simulink model "Electrical_System_2018b_obfs"  (R2019b)
settings: Solver=VariableStepAuto  StartTime=0.0  StopTime=5  RelTol=1e-3  AbsTol=1e-3  EnableMultiTasking=on
InitFcn:
  | Steady_State_Initialisation;
StopFcn:
  | %sscexplore(simlog);
  | %Logging
undefined symbols (not defined in the file): abrlhklxvp, aexgmhuedq, afmfmjnutg, afpphrjpnc, ahuxbyvruc, alarvljztt, amxnyqmnuw, aodrlwvqie, aolhmuplyq, aqpmguuqkg, auesgwirzl, aurophlnng, awamelrhru, ayfhvxflxn, azxkacuhqc, babszerikg, bawhdqanwq, bevoqecvei, bltjvqbchx, bmqsuewujl, bsmyqjfgnf, btvjbsmnve, bywgxqeadw, bziaduxaer, bzmcmdqocb, bzsvyvetat, ccsjnrbsih, cdvenygxwh, cedkrnslhx, cjheorclzs, cjrdshrtqx, ckhavyhcza, ckxewznhlz, cmrcgyiplk, conenicnws, cqkejbgjnn, csfnuwymhe, cunupkhwbh, cwzfvzuxxh, dcadmadufn, dcfponivnv, ddtrqjrhjn, dfhoxvkqas, dfrhtcwpne, dfvomcagjv, djijwylxea, dnmeqksrrm, dnzewbdkaa, dsqcykyxav, dtswwlttmm, ecumpidjtv, edegaywrct, ejjjsmnejc, eknqnehjdz, emvdetzouf, esxbqkbahr, etnkkbreiq, eunoiiiirw, ewewcuedir, fatkfxdhtc ... (+386)
libraries: fl_lib x802, ee_lib x362, fl_ps_legacy_lib x160, nesl_utility x85
(part 25 of 26)

== system Electrical_System_2018b_obfs/Redacted_1221/Redacted_7996/Redacted_1/Redacted_4377/Redacted_6082/Redacted_4413/Positive_Neutral ==
  Open Circuit : fl_lib/Electrical/Electrical Elements/Open Circuit  v_specify=off  v_priority=None  v=0 V  v_nominal_specify=off  v_nominal_unit=V  v_nominal_value=1
      settings: SourceProductName=Simscape  SourceProductBaseCode=SS
  Redacted_9976 : PMIOPort  Side=Left
  Redacted_5180 : PMIOPort  Port=2  Side=Left
  Redacted_6712 : PMIOPort  Port=3  Side=Left
  Redacted_6595 : PMIOPort  Port=4  Side=Right
  Redacted_8408 : PMIOPort  Port=5  Side=Right
  connections:
  Open Circuit/LConn1 -- Redacted_6712/RConn1
  Redacted_6595/RConn1 -- Redacted_9976/RConn1
  Redacted_5180/RConn1 -- Redacted_8408/RConn1

== system Electrical_System_2018b_obfs/Redacted_1221/Redacted_7996/Redacted_1/Redacted_4377/Redacted_6082/Redacted_4413/Redacted_6190 ==
  Redacted_6825 : fl_lib/Electrical/Electrical Elements/Open Circuit  v_specify=off  v_priority=None  v=nafaxblafc V  v_nominal_specify=off  v_nominal_unit=V  v_nominal_value=uctqgjleyg
      settings: SourceProductName=Simscape  SourceProductBaseCode=SS
  Redacted_9976 : PMIOPort  Side=Left
  Redacted_5180 : PMIOPort  Port=2  Side=Left
  Redacted_6712 : PMIOPort  Port=3  Side=Left
  Redacted_6595 : PMIOPort  Port=4  Side=Right
  Redacted_8408 : PMIOPort  Port=5  Side=Right
  connections:
  Redacted_6825/LConn1 -- Redacted_5180/RConn1
  Redacted_6595/RConn1 -- Redacted_9976/RConn1
  Redacted_8408/RConn1 -- Redacted_6712/RConn1

== system Electrical_System_2018b_obfs/Redacted_1221/Redacted_7996/Redacted_1/Redacted_4377/Redacted_6082/Redacted_5550/Neutral_Negative ==
  Open Circuit : fl_lib/Electrical/Electrical Elements/Open Circuit  v_specify=off  v_priority=None  v=0 V  v_nominal_specify=off  v_nominal_unit=V  v_nominal_value=1
      settings: SourceProductName=Simscape  SourceProductBaseCode=SS
  Redacted_6826 : PMIOPort  Side=Left
  Redacted_51 : PMIOPort  Port=2  Side=Left
  Redacted_9515 : PMIOPort  Port=3  Side=Left
  Redacted_375 : PMIOPort  Port=4  Side=Right
  Redacted_6304 : PMIOPort  Port=5  Side=Right
  connections:
  Redacted_6304/RConn1 -- Redacted_9515/RConn1
  Open Circuit/LConn1 -- Redacted_6826/RConn1
  Redacted_51/RConn1 -- Redacted_375/RConn1

== system Electrical_System_2018b_obfs/Redacted_1221/Redacted_7996/Redacted_1/Redacted_4377/Redacted_6082/Redacted_5550/Positive_Neutral ==
  Open Circuit : fl_lib/Electrical/Electrical Elements/Open Circuit  v_specify=off  v_priority=None  v=0 V  v_nominal_specify=off  v_nominal_unit=V  v_nominal_value=1
      settings: SourceProductName=Simscape  SourceProductBaseCode=SS
  Redacted_6826 : PMIOPort  Side=Left
  Redacted_51 : PMIOPort  Port=2  Side=Left
  Redacted_9515 : PMIOPort  Port=3  Side=Left
  Redacted_375 : PMIOPort  Port=4  Side=Right
  Redacted_6304 : PMIOPort  Port=5  Side=Right
  connections:
  Open Circuit/LConn1 -- Redacted_9515/RConn1
  Redacted_375/RConn1 -- Redacted_6826/RConn1
  Redacted_51/RConn1 -- Redacted_6304/RConn1

== system Electrical_System_2018b_obfs/Redacted_1221/Redacted_7996/Redacted_1/Redacted_4377/Redacted_6082/Redacted_5550/Redacted_2952 ==
  Redacted_9904 : fl_lib/Electrical/Electrical Elements/Open Circuit  v_specify=off  v_priority=None  v=cbwtykvznf V  v_nominal_specify=off  v_nominal_unit=V  v_nominal_value=bbwdbtprkb
      settings: SourceProductName=Simscape  SourceProductBaseCode=SS
  Redacted_6826 : PMIOPort  Side=Left
  Redacted_51 : PMIOPort  Port=2  Side=Left
  Redacted_9515 : PMIOPort  Port=3  Side=Left
  Redacted_375 : PMIOPort  Port=4  Side=Right
  Redacted_6304 : PMIOPort  Port=5  Side=Right
  connections:
  Redacted_9904/LConn1 -- Redacted_51/RConn1
  Redacted_375/RConn1 -- Redacted_6826/RConn1
  Redacted_6304/RConn1 -- Redacted_9515/RConn1

== system Electrical_System_2018b_obfs/Redacted_1221/Redacted_7996/Redacted_1/Redacted_4377/Redacted_6082/Redacted_5713/Neutral_Negative ==
  Open Circuit : fl_lib/Electrical/Electrical Elements/Open Circuit  v_specify=off  v_priority=None  v=0 V  v_nominal_specify=off  v_nominal_unit=V  v_nominal_value=1
      settings: SourceProductName=Simscape  SourceProductBaseCode=SS
  Redacted_6138 : PMIOPort  Side=Left
  Redacted_1431 : PMIOPort  Port=2  Side=Left
  Redacted_7946 : PMIOPort  Port=3  Side=Left
  Redacted_819 : PMIOPort  Port=4  Side=Right
  Redacted_4816 : PMIOPort  Port=5  Side=Right
  connections:
  Redacted_4816/RConn1 -- Redacted_7946/RConn1
  Open Circuit/LConn1 -- Redacted_6138/RConn1
  Redacted_1431/RConn1 -- Redacted_819/RConn1

== system Electrical_System_2018b_obfs/Redacted_1221/Redacted_7996/Redacted_1/Redacted_4377/Redacted_6082/Redacted_5713/Positive_Neutral ==
  Open Circuit : fl_lib/Electrical/Electrical Elements/Open Circuit  v_specify=off  v_priority=None  v=0 V  v_nominal_specify=off  v_nominal_unit=V  v_nominal_value=1
      settings: SourceProductName=Simscape  SourceProductBaseCode=SS
  Redacted_6138 : PMIOPort  Side=Left
  Redacted_1431 : PMIOPort  Port=2  Side=Left
  Redacted_7946 : PMIOPort  Port=3  Side=Left
  Redacted_819 : PMIOPort  Port=4  Side=Right
  Redacted_4816 : PMIOPort  Port=5  Side=Right
  connections:
  Open Circuit/LConn1 -- Redacted_7946/RConn1
  Redacted_819/RConn1 -- Redacted_6138/RConn1
  Redacted_1431/RConn1 -- Redacted_4816/RConn1

== system Electrical_System_2018b_obfs/Redacted_1221/Redacted_7996/Redacted_1/Redacted_4377/Redacted_6082/Redacted_5713/Redacted_1184 ==
  Redacted_2299 : fl_lib/Electrical/Electrical Elements/Open Circuit  v_specify=off  v_priority=None  v=tqpmitufxi V  v_nominal_specify=off  v_nominal_unit=V  v_nominal_value=nizvadugds
      settings: SourceProductName=Simscape  SourceProductBaseCode=SS
  Redacted_6138 : PMIOPort  Side=Left
  Redacted_1431 : PMIOPort  Port=2  Side=Left
  Redacted_7946 : PMIOPort  Port=3  Side=Left
  Redacted_819 : PMIOPort  Port=4  Side=Right
  Redacted_4816 : PMIOPort  Port=5  Side=Right
  connections:
  Redacted_2299/LConn1 -- Redacted_1431/RConn1
  Redacted_819/RConn1 -- Redacted_6138/RConn1
  Redacted_4816/RConn1 -- Redacted_7946/RConn1

== system Electrical_System_2018b_obfs/Redacted_1221/Redacted_7996/Redacted_1/Redacted_4377/Redacted_6082/Redacted_5976/Neutral_Negative ==
  Open Circuit : fl_lib/Electrical/Electrical Elements/Open Circuit  v_specify=off  v_priority=None  v=0 V  v_nominal_specify=off  v_nominal_unit=V  v_nominal_value=1
      settings: SourceProductName=Simscape  SourceProductBaseCode=SS
  Redacted_9241 : PMIOPort  Side=Left
  Redacted_5276 : PMIOPort  Port=2  Side=Left
  Redacted_2400 : PMIOPort  Port=3  Side=Left
  Redacted_5406 : PMIOPort  Port=4  Side=Right
  Redacted_1074 : PMIOPort  Port=5  Side=Right
  connections:
  Redacted_5276/RConn1 -- Redacted_5406/RConn1
  Open Circuit/LConn1 -- Redacted_9241/RConn1
  Redacted_1074/RConn1 -- Redacted_2400/RConn1

== system Electrical_System_2018b_obfs/Redacted_1221/Redacted_7996/Redacted_1/Redacted_4377/Redacted_6082/Redacted_5976/Positive_Neutral ==
  Open Circuit : fl_lib/Electrical/Electrical Elements/Open Circuit  v_specify=off  v_priority=None  v=0 V  v_nominal_specify=off  v_nominal_unit=V  v_nominal_value=1
      settings: SourceProductName=Simscape  SourceProductBaseCode=SS
  Redacted_9241 : PMIOPort  Side=Left
  Redacted_5276 : PMIOPort  Port=2  Side=Left
  Redacted_2400 : PMIOPort  Port=3  Side=Left
  Redacted_5406 : PMIOPort  Port=4  Side=Right
  Redacted_1074 : PMIOPort  Port=5  Side=Right
  connections:
  Redacted_5276/RConn1 -- Redacted_1074/RConn1
  Redacted_5406/RConn1 -- Redacted_9241/RConn1
  Open Circuit/LConn1 -- Redacted_2400/RConn1

== system Electrical_System_2018b_obfs/Redacted_1221/Redacted_7996/Redacted_1/Redacted_4377/Redacted_6082/Redacted_5976/Redacted_5620 ==
  Redacted_9178 : fl_lib/Electrical/Electrical Elements/Open Circuit  v_specify=off  v_priority=None  v=jhtpowznxh V  v_nominal_specify=off  v_nominal_unit=V  v_nominal_value=mubuuhzqmu
      settings: SourceProductName=Simscape  SourceProductBaseCode=SS
  Redacted_9241 : PMIOPort  Side=Left
  Redacted_5276 : PMIOPort  Port=2  Side=Left
  Redacted_2400 : PMIOPort  Port=3  Side=Left
  Redacted_5406 : PMIOPort  Port=4  Side=Right
  Redacted_1074 : PMIOPort  Port=5  Side=Right
  connections:
  Redacted_1074/RConn1 -- Redacted_2400/RConn1
  Redacted_5406/RConn1 -- Redacted_9241/RConn1
  Redacted_9178/LConn1 -- Redacted_5276/RConn1

== system Electrical_System_2018b_obfs/Redacted_1221/Redacted_7996/Redacted_1/Redacted_4377/Redacted_6082/Redacted_6424/Neutral_Negative ==
  Open Circuit : fl_lib/Electrical/Electrical Elements/Open Circuit  v_specify=off  v_priority=None  v=0 V  v_nominal_specify=off  v_nominal_unit=V  v_nominal_value=1
      settings: SourceProductName=Simscape  SourceProductBaseCode=SS
  Redacted_4582 : PMIOPort  Side=Left
  Redacted_1544 : PMIOPort  Port=2  Side=Left
  Redacted_1581 : PMIOPort  Port=3  Side=Left
  Redacted_1961 : PMIOPort  Port=4  Side=Right
  Redacted_7479 : PMIOPort  Port=5  Side=Right
  connections:
  Redacted_7479/RConn1 -- Redacted_1581/RConn1
  Open Circuit/LConn1 -- Redacted_4582/RConn1
  Redacted_1544/RConn1 -- Redacted_1961/RConn1

== system Electrical_System_2018b_obfs/Redacted_1221/Redacted_7996/Redacted_1/Redacted_4377/Redacted_6082/Redacted_6424/Positive_Neutral ==
  Open Circuit : fl_lib/Electrical/Electrical Elements/Open Circuit  v_specify=off  v_priority=None  v=0 V  v_nominal_specify=off  v_nominal_unit=V  v_nominal_value=1
      settings: SourceProductName=Simscape  SourceProductBaseCode=SS
  Redacted_4582 : PMIOPort  Side=Left
  Redacted_1544 : PMIOPort  Port=2  Side=Left
  Redacted_1581 : PMIOPort  Port=3  Side=Left
  Redacted_1961 : PMIOPort  Port=4  Side=Right
  Redacted_7479 : PMIOPort  Port=5  Side=Right
  connections:
  Open Circuit/LConn1 -- Redacted_1581/RConn1
  Redacted_1961/RConn1 -- Redacted_4582/RConn1
  Redacted_1544/RConn1 -- Redacted_7479/RConn1

== system Electrical_System_2018b_obfs/Redacted_1221/Redacted_7996/Redacted_1/Redacted_4377/Redacted_6082/Redacted_6424/Redacted_7805 ==
  Redacted_3936 : fl_lib/Electrical/Electrical Elements/Open Circuit  v_specify=off  v_priority=None  v=fjoxglgvhp V  v_nominal_specify=off  v_nominal_unit=V  v_nominal_value=omyuclhrqc
      settings: SourceProductName=Simscape  SourceProductBaseCode=SS
  Redacted_4582 : PMIOPort  Side=Left
  Redacted_1544 : PMIOPort  Port=2  Side=Left
  Redacted_1581 : PMIOPort  Port=3  Side=Left
  Redacted_1961 : PMIOPort  Port=4  Side=Right
  Redacted_7479 : PMIOPort  Port=5  Side=Right
  connections:
  Redacted_3936/LConn1 -- Redacted_1544/RConn1
  Redacted_1961/RConn1 -- Redacted_4582/RConn1
  Redacted_7479/RConn1 -- Redacted_1581/RConn1

== system Electrical_System_2018b_obfs/Redacted_1221/Redacted_7996/Redacted_1/Redacted_4377/Redacted_6082/Redacted_7051/Neutral_Negative ==
  Open Circuit : fl_lib/Electrical/Electrical Elements/Open Circuit  v_specify=off  v_priority=None  v=0 V  v_nominal_specify=off  v_nominal_unit=V  v_nominal_value=1
      settings: SourceProductName=Simscape  SourceProductBaseCode=SS
  Redacted_2697 : PMIOPort  Side=Left
  Redacted_1518 : PMIOPort  Port=2  Side=Left
  Redacted_2395 : PMIOPort  Port=3  Side=Left
  Redacted_3537 : PMIOPort  Port=4  Side=Right
  Redacted_8383 : PMIOPort  Port=5  Side=Right
  connections:
  Redacted_1518/RConn1 -- Redacted_3537/RConn1
  Open Circuit/LConn1 -- Redacted_2697/RConn1
  Redacted_8383/RConn1 -- Redacted_2395/RConn1

== system Electrical_System_2018b_obfs/Redacted_1221/Redacted_7996/Redacted_1/Redacted_4377/Redacted_6082/Redacted_7051/Positive_Neutral ==
  Open Circuit : fl_lib/Electrical/Electrical Elements/Open Circuit  v_specify=off  v_priority=None  v=0 V  v_nominal_specify=off  v_nominal_unit=V  v_nominal_value=1
      settings: SourceProductName=Simscape  SourceProductBaseCode=SS
  Redacted_2697 : PMIOPort  Side=Left
  Redacted_1518 : PMIOPort  Port=2  Side=Left
  Redacted_2395 : PMIOPort  Port=3  Side=Left
  Redacted_3537 : PMIOPort  Port=4  Side=Right
  Redacted_8383 : PMIOPort  Port=5  Side=Right
  connections:
  Redacted_1518/RConn1 -- Redacted_8383/RConn1
  Redacted_3537/RConn1 -- Redacted_2697/RConn1
  Open Circuit/LConn1 -- Redacted_2395/RConn1

== system Electrical_System_2018b_obfs/Redacted_1221/Redacted_7996/Redacted_1/Redacted_4377/Redacted_6082/Redacted_7051/Redacted_1021 ==
  Redacted_3666 : fl_lib/Electrical/Electrical Elements/Open Circuit  v_specify=off  v_priority=None  v=jitpzdpdri V  v_nominal_specify=off  v_nominal_unit=V  v_nominal_value=zhywmqlonq
      settings: SourceProductName=Simscape  SourceProductBaseCode=SS
  Redacted_2697 : PMIOPort  Side=Left
  Redacted_1518 : PMIOPort  Port=2  Side=Left
  Redacted_2395 : PMIOPort  Port=3  Side=Left
  Redacted_3537 : PMIOPort  Port=4  Side=Right
  Redacted_8383 : PMIOPort  Port=5  Side=Right
  connections:
  Redacted_8383/RConn1 -- Redacted_2395/RConn1
  Redacted_3537/RConn1 -- Redacted_2697/RConn1
  Redacted_3666/LConn1 -- Redacted_1518/RConn1

== system Electrical_System_2018b_obfs/Redacted_1221/Redacted_7996/Redacted_1/Redacted_4377/Redacted_6082/Redacted_7884/Neutral_Negative ==
  Open Circuit : fl_lib/Electrical/Electrical Elements/Open Circuit  v_specify=off  v_priority=None  v=0 V  v_nominal_specify=off  v_nominal_unit=V  v_nominal_value=1
      settings: SourceProductName=Simscape  SourceProductBaseCode=SS
  Redacted_6224 : PMIOPort  Side=Left
  Redacted_4321 : PMIOPort  Port=2  Side=Left
  Redacted_2243 : PMIOPort  Port=3  Side=Left
  Redacted_707 : PMIOPort  Port=4  Side=Right
  Redacted_8636 : PMIOPort  Port=5  Side=Right
  connections:
  Redacted_4321/RConn1 -- Redacted_707/RConn1
  Open Circuit/LConn1 -- Redacted_6224/RConn1
  Redacted_8636/RConn1 -- Redacted_2243/RConn1

== system Electrical_System_2018b_obfs/Redacted_1221/Redacted_7996/Redacted_1/Redacted_4377/Redacted_6082/Redacted_7884/Positive_Neutral ==
  Open Circuit : fl_lib/Electrical/Electrical Elements/Open Circuit  v_specify=off  v_priority=None  v=0 V  v_nominal_specify=off  v_nominal_unit=V  v_nominal_value=1
      settings: SourceProductName=Simscape  SourceProductBaseCode=SS
  Redacted_6224 : PMIOPort  Side=Left
  Redacted_4321 : PMIOPort  Port=2  Side=Left
  Redacted_2243 : PMIOPort  Port=3  Side=Left
  Redacted_707 : PMIOPort  Port=4  Side=Right
  Redacted_8636 : PMIOPort  Port=5  Side=Right
  connections:
  Redacted_4321/RConn1 -- Redacted_8636/RConn1
  Redacted_707/RConn1 -- Redacted_6224/RConn1
  Open Circuit/LConn1 -- Redacted_2243/RConn1

== system Electrical_System_2018b_obfs/Redacted_1221/Redacted_7996/Redacted_1/Redacted_4377/Redacted_6082/Redacted_7884/Redacted_81 ==
  Redacted_8822 : fl_lib/Electrical/Electrical Elements/Open Circuit  v_specify=off  v_priority=None  v=nrbmgkomdb V  v_nominal_specify=off  v_nominal_unit=V  v_nominal_value=chrfcotgkg
      settings: SourceProductName=Simscape  SourceProductBaseCode=SS
  Redacted_6224 : PMIOPort  Side=Left
  Redacted_4321 : PMIOPort  Port=2  Side=Left
  Redacted_2243 : PMIOPort  Port=3  Side=Left
  Redacted_707 : PMIOPort  Port=4  Side=Right
  Redacted_8636 : PMIOPort  Port=5  Side=Right
  connections:
  Redacted_8636/RConn1 -- Redacted_2243/RConn1
  Redacted_707/RConn1 -- Redacted_6224/RConn1
  Redacted_8822/LConn1 -- Redacted_4321/RConn1

== system Electrical_System_2018b_obfs/Redacted_1221/Redacted_7996/Redacted_1/Redacted_4377/Redacted_6082/Redacted_8502/Neutral_Negative ==
  Open Circuit : fl_lib/Electrical/Electrical Elements/Open Circuit  v_specify=off  v_priority=None  v=0 V  v_nominal_specify=off  v_nominal_unit=V  v_nominal_value=1
      settings: SourceProductName=Simscape  SourceProductBaseCode=SS
  Redacted_389 : PMIOPort  Side=Left
  Redacted_6488 : PMIOPort  Port=2  Side=Left
  Redacted_5156 : PMIOPort  Port=3  Side=Left
  Redacted_180 : PMIOPort  Port=4  Side=Right
  Redacted_7018 : PMIOPort  Port=5  Side=Right
  connections:
  Redacted_6488/RConn1 -- Redacted_180/RConn1
  Open Circuit/LConn1 -- Redacted_389/RConn1
  Redacted_7018/RConn1 -- Redacted_5156/RConn1

== system Electrical_System_2018b_obfs/Redacted_1221/Redacted_7996/Redacted_1/Redacted_4377/Redacted_6082/Redacted_8502/Positive_Neutral ==
  Open Circuit : fl_lib/Electrical/Electrical Elements/Open Circuit  v_specify=off  v_priority=None  v=0 V  v_nominal_specify=off  v_nominal_unit=V  v_nominal_value=1
      settings: SourceProductName=Simscape  SourceProductBaseCode=SS
  Redacted_389 : PMIOPort  Side=Left
  Redacted_6488 : PMIOPort  Port=2  Side=Left
  Redacted_5156 : PMIOPort  Port=3  Side=Left
  Redacted_180 : PMIOPort  Port=4  Side=Right
  Redacted_7018 : PMIOPort  Port=5  Side=Right
  connections:
  Redacted_6488/RConn1 -- Redacted_7018/RConn1
  Redacted_180/RConn1 -- Redacted_389/RConn1
  Open Circuit/LConn1 -- Redacted_5156/RConn1

== system Electrical_System_2018b_obfs/Redacted_1221/Redacted_7996/Redacted_1/Redacted_4377/Redacted_6082/Redacted_8502/Redacted_4068 ==
  Redacted_9772 : fl_lib/Electrical/Electrical Elements/Open Circuit  v_specify=off  v_priority=None  v=truhycjrml V  v_nominal_specify=off  v_nominal_unit=V  v_nominal_value=fuzhyyoiey
      settings: SourceProductName=Simscape  SourceProductBaseCode=SS
  Redacted_389 : PMIOPort  Side=Left
  Redacted_6488 : PMIOPort  Port=2  Side=Left
  Redacted_5156 : PMIOPort  Port=3  Side=Left
  Redacted_180 : PMIOPort  Port=4  Side=Right
  Redacted_7018 : PMIOPort  Port=5  Side=Right
  connections:
  Redacted_7018/RConn1 -- Redacted_5156/RConn1
  Redacted_180/RConn1 -- Redacted_389/RConn1
  Redacted_9772/LConn1 -- Redacted_6488/RConn1

== system Electrical_System_2018b_obfs/Redacted_1221/Redacted_7996/Redacted_1/Redacted_4377/Redacted_6082/Redacted_9034/Neutral_Negative ==
  Open Circuit : fl_lib/Electrical/Electrical Elements/Open Circuit  v_specify=off  v_priority=None  v=0 V  v_nominal_specify=off  v_nominal_unit=V  v_nominal_value=1
      settings: SourceProductName=Simscape  SourceProductBaseCode=SS
  Redacted_4887 : PMIOPort  Side=Left
  Redacted_5529 : PMIOPort  Port=2  Side=Left
  Redacted_4069 : PMIOPort  Port=3  Side=Left
  Redacted_1826 : PMIOPort  Port=4  Side=Right
  Redacted_1222 : PMIOPort  Port=5  Side=Right
  connections:
  Redacted_1222/RConn1 -- Redacted_4069/RConn1
  Open Circuit/LConn1 -- Redacted_4887/RConn1
  Redacted_5529/RConn1 -- Redacted_1826/RConn1

== system Electrical_System_2018b_obfs/Redacted_1221/Redacted_7996/Redacted_1/Redacted_4377/Redacted_6082/Redacted_9034/Positive_Neutral ==
  Open Circuit : fl_lib/Electrical/Electrical Elements/Open Circuit  v_specify=off  v_priority=None  v=0 V  v_nominal_specify=off  v_nominal_unit=V  v_nominal_value=1
      settings: SourceProductName=Simscape  SourceProductBaseCode=SS
  Redacted_4887 : PMIOPort  Side=Left
  Redacted_5529 : PMIOPort  Port=2  Side=Left
  Redacted_4069 : PMIOPort  Port=3  Side=Left
  Redacted_1826 : PMIOPort  Port=4  Side=Right
  Redacted_1222 : PMIOPort  Port=5  Side=Right
  connections:
  Open Circuit/LConn1 -- Redacted_4069/RConn1
  Redacted_1826/RConn1 -- Redacted_4887/RConn1
  Redacted_5529/RConn1 -- Redacted_1222/RConn1

== system Electrical_System_2018b_obfs/Redacted_1221/Redacted_7996/Redacted_1/Redacted_4377/Redacted_6082/Redacted_9034/Redacted_4182 ==
  Redacted_1436 : fl_lib/Electrical/Electrical Elements/Open Circuit  v_specify=off  v_priority=None  v=zzrofiuybt V  v_nominal_specify=off  v_nominal_unit=V  v_nominal_value=ignlzzzuid
      settings: SourceProductName=Simscape  SourceProductBaseCode=SS
  Redacted_4887 : PMIOPort  Side=Left
  Redacted_5529 : PMIOPort  Port=2  Side=Left
  Redacted_4069 : PMIOPort  Port=3  Side=Left
  Redacted_1826 : PMIOPort  Port=4  Side=Right
  Redacted_1222 : PMIOPort  Port=5  Side=Right
  connections:
  Redacted_1436/LConn1 -- Redacted_5529/RConn1
  Redacted_1826/RConn1 -- Redacted_4887/RConn1
  Redacted_1222/RConn1 -- Redacted_4069/RConn1

== system Electrical_System_2018b_obfs/Redacted_1221/Redacted_7996/Redacted_1/Redacted_4377/Redacted_6082/Redacted_9572/Neutral_Negative ==
  Open Circuit : fl_lib/Electrical/Electrical Elements/Open Circuit  v_specify=off  v_priority=None  v=0 V  v_nominal_specify=off  v_nominal_unit=V  v_nominal_value=1
      settings: SourceProductName=Simscape  SourceProductBaseCode=SS
  Redacted_435 : PMIOPort  Side=Left
  Redacted_1376 : PMIOPort  Port=2  Side=Left
  Redacted_8237 : PMIOPort  Port=3  Side=Left
  Redacted_4941 : PMIOPort  Port=4  Side=Right
  Redacted_729 : PMIOPort  Port=5  Side=Right
  connections:
  Redacted_1376/RConn1 -- Redacted_4941/RConn1
  Open Circuit/LConn1 -- Redacted_435/RConn1
  Redacted_729/RConn1 -- Redacted_8237/RConn1

== system Electrical_System_2018b_obfs/Redacted_1221/Redacted_7996/Redacted_1/Redacted_4377/Redacted_6082/Redacted_9572/Positive_Neutral ==
  Open Circuit : fl_lib/Electrical/Electrical Elements/Open Circuit  v_specify=off  v_priority=None  v=0 V  v_nominal_specify=off  v_nominal_unit=V  v_nominal_value=1
      settings: SourceProductName=Simscape  SourceProductBaseCode=SS
  Redacted_435 : PMIOPort  Side=Left
  Redacted_1376 : PMIOPort  Port=2  Side=Left
  Redacted_8237 : PMIOPort  Port=3  Side=Left
  Redacted_4941 : PMIOPort  Port=4  Side=Right
  Redacted_729 : PMIOPort  Port=5  Side=Right
  connections:
  Redacted_1376/RConn1 -- Redacted_729/RConn1
  Redacted_4941/RConn1 -- Redacted_435/RConn1
  Open Circuit/LConn1 -- Redacted_8237/RConn1

== system Electrical_System_2018b_obfs/Redacted_1221/Redacted_7996/Redacted_1/Redacted_4377/Redacted_6082/Redacted_9572/Redacted_3288 ==
  Redacted_4505 : fl_lib/Electrical/Electrical Elements/Open Circuit  v_specify=off  v_priority=None  v=bjybeoqvmc V  v_nominal_specify=off  v_nominal_unit=V  v_nominal_value=ldxcbaigcw
      settings: SourceProductName=Simscape  SourceProductBaseCode=SS
  Redacted_435 : PMIOPort  Side=Left
  Redacted_1376 : PMIOPort  Port=2  Side=Left
  Redacted_8237 : PMIOPort  Port=3  Side=Left
  Redacted_4941 : PMIOPort  Port=4  Side=Right
  Redacted_729 : PMIOPort  Port=5  Side=Right
  connections:
  Redacted_729/RConn1 -- Redacted_8237/RConn1
  Redacted_4941/RConn1 -- Redacted_435/RConn1
  Redacted_4505/LConn1 -- Redacted_1376/RConn1

== system Electrical_System_2018b_obfs/Redacted_1221/Redacted_7996/Redacted_1/Redacted_4377/Redacted_6082/Redacted_980/Neutral_Negative ==
  Open Circuit : fl_lib/Electrical/Electrical Elements/Open Circuit  v_specify=off  v_priority=None  v=0 V  v_nominal_specify=off  v_nominal_unit=V  v_nominal_value=1
      settings: SourceProductName=Simscape  SourceProductBaseCode=SS
  Redacted_3281 : PMIOPort  Side=Left
  Redacted_9175 : PMIOPort  Port=2  Side=Left
  Redacted_1087 : PMIOPort  Port=3  Side=Left
  Redacted_2672 : PMIOPort  Port=4  Side=Right
  Redacted_3599 : PMIOPort  Port=5  Side=Right
  connections:
  Redacted_3599/RConn1 -- Redacted_1087/RConn1
  Open Circuit/LConn1 -- Redacted_3281/RConn1
  Redacted_9175/RConn1 -- Redacted_2672/RConn1

== system Electrical_System_2018b_obfs/Redacted_1221/Redacted_7996/Redacted_1/Redacted_4377/Redacted_6082/Redacted_980/Positive_Neutral ==
  Open Circuit : fl_lib/Electrical/Electrical Elements/Open Circuit  v_specify=off  v_priority=None  v=0 V  v_nominal_specify=off  v_nominal_unit=V  v_nominal_value=1
      settings: SourceProductName=Simscape  SourceProductBaseCode=SS
  Redacted_3281 : PMIOPort  Side=Left
  Redacted_9175 : PMIOPort  Port=2  Side=Left
  Redacted_1087 : PMIOPort  Port=3  Side=Left
  Redacted_2672 : PMIOPort  Port=4  Side=Right
  Redacted_3599 : PMIOPort  Port=5  Side=Right
  connections:
  Open Circuit/LConn1 -- Redacted_1087/RConn1
  Redacted_2672/RConn1 -- Redacted_3281/RConn1
  Redacted_9175/RConn1 -- Redacted_3599/RConn1

== system Electrical_System_2018b_obfs/Redacted_1221/Redacted_7996/Redacted_1/Redacted_4377/Redacted_6082/Redacted_980/Redacted_8833 ==
  Redacted_4926 : fl_lib/Electrical/Electrical Elements/Open Circuit  v_specify=off  v_priority=None  v=pdiyatassn V  v_nominal_specify=off  v_nominal_unit=V  v_nominal_value=uflvhyhiqw
      settings: SourceProductName=Simscape  SourceProductBaseCode=SS
  Redacted_3281 : PMIOPort  Side=Left
  Redacted_9175 : PMIOPort  Port=2  Side=Left
  Redacted_1087 : PMIOPort  Port=3  Side=Left
  Redacted_2672 : PMIOPort  Port=4  Side=Right
  Redacted_3599 : PMIOPort  Port=5  Side=Right
  connections:
  Redacted_4926/LConn1 -- Redacted_9175/RConn1
  Redacted_2672/RConn1 -- Redacted_3281/RConn1
  Redacted_3599/RConn1 -- Redacted_1087/RConn1

== system Electrical_System_2018b_obfs/Redacted_1221/Redacted_7996/Redacted_2/Redacted_38/Redacted_8107/Redacted_3070/Neutral_Negative ==
  Open Circuit : fl_lib/Electrical/Electrical Elements/Open Circuit  v_specify=off  v_priority=None  v=0 V  v_nominal_specify=off  v_nominal_unit=V  v_nominal_value=1
      settings: SourceProductName=Simscape  SourceProductBaseCode=SS
  Redacted_9800 : PMIOPort  Side=Left
  Redacted_6600 : PMIOPort  Port=2  Side=Left
  Redacted_5239 : PMIOPort  Port=3  Side=Left
  Redacted_3081 : PMIOPort  Port=4  Side=Right
  Redacted_7642 : PMIOPort  Port=5  Side=Right
  connections:
  Redacted_7642/RConn1 -- Redacted_5239/RConn1
  Open Circuit/LConn1 -- Redacted_9800/RConn1
  Redacted_6600/RConn1 -- Redacted_3081/RConn1

== system Electrical_System_2018b_obfs/Redacted_1221/Redacted_7996/Redacted_2/Redacted_38/Redacted_8107/Redacted_3070/Positive_Neutral ==
  Open Circuit : fl_lib/Electrical/Electrical Elements/Open Circuit  v_specify=off  v_priority=None  v=0 V  v_nominal_specify=off  v_nominal_unit=V  v_nominal_value=1
      settings: SourceProductName=Simscape  SourceProductBaseCode=SS
  Redacted_9800 : PMIOPort  Side=Left
  Redacted_6600 : PMIOPort  Port=2  Side=Left
  Redacted_5239 : PMIOPort  Port=3  Side=Left
  Redacted_3081 : PMIOPort  Port=4  Side=Right
  Redacted_7642 : PMIOPort  Port=5  Side=Right
  connections:
  Open Circuit/LConn1 -- Redacted_5239/RConn1
  Redacted_3081/RConn1 -- Redacted_9800/RConn1
  Redacted_6600/RConn1 -- Redacted_7642/RConn1

== system Electrical_System_2018b_obfs/Redacted_1221/Redacted_7996/Redacted_2/Redacted_38/Redacted_8107/Redacted_3070/Redacted_6581 ==
  Redacted_9951 : fl_lib/Electrical/Electrical Elements/Open Circuit  v_specify=off  v_priority=None  v=kbecunztrl V  v_nominal_specify=off  v_nominal_unit=V  v_nominal_value=jkubweymaj
      settings: SourceProductName=Simscape  SourceProductBaseCode=SS
  Redacted_9800 : PMIOPort  Side=Left
  Redacted_6600 : PMIOPort  Port=2  Side=Left
  Redacted_5239 : PMIOPort  Port=3  Side=Left
  Redacted_3081 : PMIOPort  Port=4  Side=Right
  Redacted_7642 : PMIOPort  Port=5  Side=Right
  connections:
  Redacted_9951/LConn1 -- Redacted_6600/RConn1
  Redacted_3081/RConn1 -- Redacted_9800/RConn1
  Redacted_7642/RConn1 -- Redacted_5239/RConn1

== system Electrical_System_2018b_obfs/Redacted_1221/Redacted_7996/Redacted_2/Redacted_38/Redacted_8107/Redacted_8444/Neutral_Negative ==
  Open Circuit : fl_lib/Electrical/Electrical Elements/Open Circuit  v_specify=off  v_priority=None  v=0 V  v_nominal_specify=off  v_nominal_unit=V  v_nominal_value=1
      settings: SourceProductName=Simscape  SourceProductBaseCode=SS
  Redacted_8974 : PMIOPort  Side=Left
  Redacted_9727 : PMIOPort  Port=2  Side=Left
  Redacted_5818 : PMIOPort  Port=3  Side=Left
  Redacted_9930 : PMIOPort  Port=4  Side=Right
  Redacted_8840 : PMIOPort  Port=5  Side=Right
  connections:
  Redacted_9727/RConn1 -- Redacted_9930/RConn1
  Open Circuit/LConn1 -- Redacted_8974/RConn1
  Redacted_8840/RConn1 -- Redacted_5818/RConn1

== system Electrical_System_2018b_obfs/Redacted_1221/Redacted_7996/Redacted_2/Redacted_38/Redacted_8107/Redacted_8444/Positive_Neutral ==
  Open Circuit : fl_lib/Electrical/Electrical Elements/Open Circuit  v_specify=off  v_priority=None  v=0 V  v_nominal_specify=off  v_nominal_unit=V  v_nominal_value=1
      settings: SourceProductName=Simscape  SourceProductBaseCode=SS
  Redacted_8974 : PMIOPort  Side=Left
  Redacted_9727 : PMIOPort  Port=2  Side=Left
  Redacted_5818 : PMIOPort  Port=3  Side=Left
  Redacted_9930 : PMIOPort  Port=4  Side=Right
  Redacted_8840 : PMIOPort  Port=5  Side=Right
  connections:
  Redacted_9727/RConn1 -- Redacted_8840/RConn1
  Redacted_9930/RConn1 -- Redacted_8974/RConn1
  Open Circuit/LConn1 -- Redacted_5818/RConn1

== system Electrical_System_2018b_obfs/Redacted_1221/Redacted_7996/Redacted_2/Redacted_38/Redacted_8107/Redacted_8444/Redacted_3917 ==
  Redacted_1857 : fl_lib/Electrical/Electrical Elements/Open Circuit  v_specify=off  v_priority=None  v=xcvpklmsqm V  v_nominal_specify=off  v_nominal_unit=V  v_nominal_value=rzgrfophqu
      settings: SourceProductName=Simscape  SourceProductBaseCode=SS
  Redacted_8974 : PMIOPort  Side=Left
  Redacted_9727 : PMIOPort  Port=2  Side=Left
  Redacted_5818 : PMIOPort  Port=3  Side=Left
  Redacted_9930 : PMIOPort  Port=4  Side=Right
  Redacted_8840 : PMIOPort  Port=5  Side=Right
  connections:
  Redacted_8840/RConn1 -- Redacted_5818/RConn1
  Redacted_9930/RConn1 -- Redacted_8974/RConn1
  Redacted_1857/LConn1 -- Redacted_9727/RConn1

== system Electrical_System_2018b_obfs/Redacted_1221/Redacted_7996/Redacted_7418/Redacted_4377/Redacted_6082/Redacted_144/Neutral_Negative ==
  Open Circuit : fl_lib/Electrical/Electrical Elements/Open Circuit  v_specify=off  v_priority=None  v=0 V  v_nominal_specify=off  v_nominal_unit=V  v_nominal_value=1
      settings: SourceProductName=Simscape  SourceProductBaseCode=SS
  Redacted_3879 : PMIOPort  Side=Left
  Redacted_3368 : PMIOPort  Port=2  Side=Left
  Redacted_9451 : PMIOPort  Port=3  Side=Left
  Redacted_8432 : PMIOPort  Port=4  Side=Right
  Redacted_6806 : PMIOPort  Port=5  Side=Right
  connections:
  Redacted_6806/RConn1 -- Redacted_9451/RConn1
  Open Circuit/LConn1 -- Redacted_3879/RConn1
  Redacted_3368/RConn1 -- Redacted_8432/RConn1

== system Electrical_System_2018b_obfs/Redacted_1221/Redacted_7996/Redacted_7418/Redacted_4377/Redacted_6082/Redacted_144/Positive_Neutral ==
  Open Circuit : fl_lib/Electrical/Electrical Elements/Open Circuit  v_specify=off  v_priority=None  v=0 V  v_nominal_specify=off  v_nominal_unit=V  v_nominal_value=1
      settings: SourceProductName=Simscape  SourceProductBaseCode=SS
  Redacted_3879 : PMIOPort  Side=Left
  Redacted_3368 : PMIOPort  Port=2  Side=Left
  Redacted_9451 : PMIOPort  Port=3  Side=Left
  Redacted_8432 : PMIOPort  Port=4  Side=Right
  Redacted_6806 : PMIOPort  Port=5  Side=Right
  connections:
  Open Circuit/LConn1 -- Redacted_9451/RConn1
  Redacted_8432/RConn1 -- Redacted_3879/RConn1
  Redacted_3368/RConn1 -- Redacted_6806/RConn1

== system Electrical_System_2018b_obfs/Redacted_1221/Redacted_7996/Redacted_7418/Redacted_4377/Redacted_6082/Redacted_144/Redacted_9503 ==
  Redacted_4565 : fl_lib/Electrical/Electrical Elements/Open Circuit  v_specify=off  v_priority=None  v=skhzijqmdj V  v_nominal_specify=off  v_nominal_unit=V  v_nominal_value=jdqusxliha
      settings: SourceProductName=Simscape  SourceProductBaseCode=SS
  Redacted_3879 : PMIOPort  Side=Left
  Redacted_3368 : PMIOPort  Port=2  Side=Left
  Redacted_9451 : PMIOPort  Port=3  Side=Left
  Redacted_8432 : PMIOPort  Port=4  Side=Right
  Redacted_6806 : PMIOPort  Port=5  Side=Right
  connections:
  Redacted_4565/LConn1 -- Redacted_3368/RConn1
  Redacted_8432/RConn1 -- Redacted_3879/RConn1
  Redacted_6806/RConn1 -- Redacted_9451/RConn1

== system Electrical_System_2018b_obfs/Redacted_1221/Redacted_7996/Redacted_7418/Redacted_4377/Redacted_6082/Redacted_1544/Neutral_Negative ==
  Open Circuit : fl_lib/Electrical/Electrical Elements/Open Circuit  v_specify=off  v_priority=None  v=0 V  v_nominal_specify=off  v_nominal_unit=V  v_nominal_value=1
      settings: SourceProductName=Simscape  SourceProductBaseCode=SS
  Redacted_697 : PMIOPort  Side=Left
  Redacted_9789 : PMIOPort  Port=2  Side=Left
  Redacted_5820 : PMIOPort  Port=3  Side=Left
  Redacted_1167 : PMIOPort  Port=4  Side=Right
  Redacted_9408 : PMIOPort  Port=5  Side=Right
  connections:
  Redacted_9408/RConn1 -- Redacted_5820/RConn1
  Open Circuit/LConn1 -- Redacted_697/RConn1
  Redacted_9789/RConn1 -- Redacted_1167/RConn1

== system Electrical_System_2018b_obfs/Redacted_1221/Redacted_7996/Redacted_7418/Redacted_4377/Redacted_6082/Redacted_1544/Positive_Neutral ==
  Open Circuit : fl_lib/Electrical/Electrical Elements/Open Circuit  v_specify=off  v_priority=None  v=0 V  v_nominal_specify=off  v_nominal_unit=V  v_nominal_value=1
      settings: SourceProductName=Simscape  SourceProductBaseCode=SS
  Redacted_697 : PMIOPort  Side=Left
  Redacted_9789 : PMIOPort  Port=2  Side=Left
  Redacted_5820 : PMIOPort  Port=3  Side=Left
  Redacted_1167 : PMIOPort  Port=4  Side=Right
  Redacted_9408 : PMIOPort  Port=5  Side=Right
  connections:
  Open Circuit/LConn1 -- Redacted_5820/RConn1
  Redacted_1167/RConn1 -- Redacted_697/RConn1
  Redacted_9789/RConn1 -- Redacted_9408/RConn1

== system Electrical_System_2018b_obfs/Redacted_1221/Redacted_7996/Redacted_7418/Redacted_4377/Redacted_6082/Redacted_1544/Redacted_4672 ==
  Redacted_7052 : fl_lib/Electrical/Electrical Elements/Open Circuit  v_specify=off  v_priority=None  v=fpovqwbuex V  v_nominal_specify=off  v_nominal_unit=V  v_nominal_value=qdnyfekgsz
      settings: SourceProductName=Simscape  SourceProductBaseCode=SS
  Redacted_697 : PMIOPort  Side=Left
  Redacted_9789 : PMIOPort  Port=2  Side=Left
  Redacted_5820 : PMIOPort  Port=3  Side=Left
  Redacted_1167 : PMIOPort  Port=4  Side=Right
  Redacted_9408 : PMIOPort  Port=5  Side=Right
  connections:
  Redacted_7052/LConn1 -- Redacted_9789/RConn1
  Redacted_1167/RConn1 -- Redacted_697/RConn1
  Redacted_9408/RConn1 -- Redacted_5820/RConn1

== system Electrical_System_2018b_obfs/Redacted_1221/Redacted_7996/Redacted_7418/Redacted_4377/Redacted_6082/Redacted_1843/Neutral_Negative ==
  Open Circuit : fl_lib/Electrical/Electrical Elements/Open Circuit  v_specify=off  v_priority=None  v=0 V  v_nominal_specify=off  v_nominal_unit=V  v_nominal_value=1
      settings: SourceProductName=Simscape  SourceProductBaseCode=SS
  Redacted_2601 : PMIOPort  Side=Left
  Redacted_5367 : PMIOPort  Port=2  Side=Left
  Redacted_1109 : PMIOPort  Port=3  Side=Left
  Redacted_4235 : PMIOPort  Port=4  Side=Right
  Redacted_9086 : PMIOPort  Port=5  Side=Right
  connections:
  Redacted_5367/RConn1 -- Redacted_4235/RConn1
  Open Circuit/LConn1 -- Redacted_2601/RConn1
  Redacted_9086/RConn1 -- Redacted_1109/RConn1

== system Electrical_System_2018b_obfs/Redacted_1221/Redacted_7996/Redacted_7418/Redacted_4377/Redacted_6082/Redacted_1843/Positive_Neutral ==
  Open Circuit : fl_lib/Electrical/Electrical Elements/Open Circuit  v_specify=off  v_priority=None  v=0 V  v_nominal_specify=off  v_nominal_unit=V  v_nominal_value=1
      settings: SourceProductName=Simscape  SourceProductBaseCode=SS
  Redacted_2601 : PMIOPort  Side=Left
  Redacted_5367 : PMIOPort  Port=2  Side=Left
  Redacted_1109 : PMIOPort  Port=3  Side=Left
  Redacted_4235 : PMIOPort  Port=4  Side=Right
  Redacted_9086 : PMIOPort  Port=5  Side=Right
  connections:
  Redacted_5367/RConn1 -- Redacted_9086/RConn1
  Redacted_4235/RConn1 -- Redacted_2601/RConn1
  Open Circuit/LConn1 -- Redacted_1109/RConn1

== system Electrical_System_2018b_obfs/Redacted_1221/Redacted_7996/Redacted_7418/Redacted_4377/Redacted_6082/Redacted_1843/Redacted_8971 ==
  Redacted_4113 : fl_lib/Electrical/Electrical Elements/Open Circuit  v_specify=off  v_priority=None  v=zogltdvlrz V  v_nominal_specify=off  v_nominal_unit=V  v_nominal_value=pakbffiyvg
      settings: SourceProductName=Simscape  SourceProductBaseCode=SS
  Redacted_2601 : PMIOPort  Side=Left
  Redacted_5367 : PMIOPort  Port=2  Side=Left
  Redacted_1109 : PMIOPort  Port=3  Side=Left
  Redacted_4235 : PMIOPort  Port=4  Side=Right
  Redacted_9086 : PMIOPort  Port=5  Side=Right
  connections:
  Redacted_9086/RConn1 -- Redacted_1109/RConn1
  Redacted_4235/RConn1 -- Redacted_2601/RConn1
  Redacted_4113/LConn1 -- Redacted_5367/RConn1

== system Electrical_System_2018b_obfs/Redacted_1221/Redacted_7996/Redacted_7418/Redacted_4377/Redacted_6082/Redacted_2005/Neutral_Negative ==
  Open Circuit : fl_lib/Electrical/Electrical Elements/Open Circuit  v_specify=off  v_priority=None  v=0 V  v_nominal_specify=off  v_nominal_unit=V  v_nominal_value=1
      settings: SourceProductName=Simscape  SourceProductBaseCode=SS
  Redacted_8266 : PMIOPort  Side=Left
  Redacted_1423 : PMIOPort  Port=2  Side=Left
  Redacted_7633 : PMIOPort  Port=3  Side=Left
  Redacted_8552 : PMIOPort  Port=4  Side=Right
  Redacted_2441 : PMIOPort  Port=5  Side=Right
  connections:
  Redacted_1423/RConn1 -- Redacted_8552/RConn1
  Open Circuit/LConn1 -- Redacted_8266/RConn1
  Redacted_2441/RConn1 -- Redacted_7633/RConn1

== system Electrical_System_2018b_obfs/Redacted_1221/Redacted_7996/Redacted_7418/Redacted_4377/Redacted_6082/Redacted_2005/Positive_Neutral ==
  Open Circuit : fl_lib/Electrical/Electrical Elements/Open Circuit  v_specify=off  v_priority=None  v=0 V  v_nominal_specify=off  v_nominal_unit=V  v_nominal_value=1
      settings: SourceProductName=Simscape  SourceProductBaseCode=SS
  Redacted_8266 : PMIOPort  Side=Left
  Redacted_1423 : PMIOPort  Port=2  Side=Left
  Redacted_7633 : PMIOPort  Port=3  Side=Left
  Redacted_8552 : PMIOPort  Port=4  Side=Right
  Redacted_2441 : PMIOPort  Port=5  Side=Right
  connections:
  Redacted_1423/RConn1 -- Redacted_2441/RConn1
  Redacted_8552/RConn1 -- Redacted_8266/RConn1
  Open Circuit/LConn1 -- Redacted_7633/RConn1

== system Electrical_System_2018b_obfs/Redacted_1221/Redacted_7996/Redacted_7418/Redacted_4377/Redacted_6082/Redacted_2005/Redacted_335 ==
  Redacted_2493 : fl_lib/Electrical/Electrical Elements/Open Circuit  v_specify=off  v_priority=None  v=wmavnefycp V  v_nominal_specify=off  v_nominal_unit=V  v_nominal_value=nysfzchmom
      settings: SourceProductName=Simscape  SourceProductBaseCode=SS
  Redacted_8266 : PMIOPort  Side=Left
  Redacted_1423 : PMIOPort  Port=2  Side=Left
  Redacted_7633 : PMIOPort  Port=3  Side=Left
  Redacted_8552 : PMIOPort  Port=4  Side=Right
  Redacted_2441 : PMIOPort  Port=5  Side=Right
  connections:
  Redacted_2441/RConn1 -- Redacted_7633/RConn1
  Redacted_8552/RConn1 -- Redacted_8266/RConn1
  Redacted_2493/LConn1 -- Redacted_1423/RConn1

== system Electrical_System_2018b_obfs/Redacted_1221/Redacted_7996/Redacted_7418/Redacted_4377/Redacted_6082/Redacted_2122/Neutral_Negative ==
  Open Circuit : fl_lib/Electrical/Electrical Elements/Open Circuit  v_specify=off  v_priority=None  v=0 V  v_nominal_specify=off  v_nominal_unit=V  v_nominal_value=1
      settings: SourceProductName=Simscape  SourceProductBaseCode=SS
  Redacted_659 : PMIOPort  Side=Left
  Redacted_1619 : PMIOPort  Port=2  Side=Left
  Redacted_5171 : PMIOPort  Port=3  Side=Left
  Redacted_2219 : PMIOPort  Port=4  Side=Right
  Redacted_5591 : PMIOPort  Port=5  Side=Right
  connections:
  Redacted_1619/RConn1 -- Redacted_2219/RConn1
  Open Circuit/LConn1 -- Redacted_659/RConn1
  Redacted_5591/RConn1 -- Redacted_5171/RConn1

== system Electrical_System_2018b_obfs/Redacted_1221/Redacted_7996/Redacted_7418/Redacted_4377/Redacted_6082/Redacted_2122/Positive_Neutral ==
  Open Circuit : fl_lib/Electrical/Electrical Elements/Open Circuit  v_specify=off  v_priority=None  v=0 V  v_nominal_specify=off  v_nominal_unit=V  v_nominal_value=1
      settings: SourceProductName=Simscape  SourceProductBaseCode=SS
  Redacted_659 : PMIOPort  Side=Left
  Redacted_1619 : PMIOPort  Port=2  Side=Left
  Redacted_5171 : PMIOPort  Port=3  Side=Left
  Redacted_2219 : PMIOPort  Port=4  Side=Right
  Redacted_5591 : PMIOPort  Port=5  Side=Right
  connections:
  Redacted_1619/RConn1 -- Redacted_5591/RConn1
  Redacted_2219/RConn1 -- Redacted_659/RConn1
  Open Circuit/LConn1 -- Redacted_5171/RConn1

== system Electrical_System_2018b_obfs/Redacted_1221/Redacted_7996/Redacted_7418/Redacted_4377/Redacted_6082/Redacted_2122/Redacted_1391 ==
  Redacted_2352 : fl_lib/Electrical/Electrical Elements/Open Circuit  v_specify=off  v_priority=None  v=jgljlridlh V  v_nominal_specify=off  v_nominal_unit=V  v_nominal_value=owhqxwlzxm
      settings: SourceProductName=Simscape  SourceProductBaseCode=SS
  Redacted_659 : PMIOPort  Side=Left
  Redacted_1619 : PMIOPort  Port=2  Side=Left
  Redacted_5171 : PMIOPort  Port=3  Side=Left
  Redacted_2219 : PMIOPort  Port=4  Side=Right
  Redacted_5591 : PMIOPort  Port=5  Side=Right
  connections:
  Redacted_5591/RConn1 -- Redacted_5171/RConn1
  Redacted_2219/RConn1 -- Redacted_659/RConn1
  Redacted_2352/LConn1 -- Redacted_1619/RConn1

== system Electrical_System_2018b_obfs/Redacted_1221/Redacted_7996/Redacted_7418/Redacted_4377/Redacted_6082/Redacted_2443/Neutral_Negative ==
  Open Circuit : fl_lib/Electrical/Electrical Elements/Open Circuit  v_specify=off  v_priority=None  v=0 V  v_nominal_specify=off  v_nominal_unit=V  v_nominal_value=1
      settings: SourceProductName=Simscape  SourceProductBaseCode=SS
  Redacted_2078 : PMIOPort  Side=Left
  Redacted_827 : PMIOPort  Port=2  Side=Left
  Redacted_65 : PMIOPort  Port=3  Side=Left
  Redacted_2555 : PMIOPort  Port=4  Side=Right
  Redacted_7416 : PMIOPort  Port=5  Side=Right
  connections:
  Redacted_827/RConn1 -- Redacted_2555/RConn1
  Open Circuit/LConn1 -- Redacted_2078/RConn1
  Redacted_7416/RConn1 -- Redacted_65/RConn1

== system Electrical_System_2018b_obfs/Redacted_1221/Redacted_7996/Redacted_7418/Redacted_4377/Redacted_6082/Redacted_2443/Positive_Neutral ==
  Open Circuit : fl_lib/Electrical/Electrical Elements/Open Circuit  v_specify=off  v_priority=None  v=0 V  v_nominal_specify=off  v_nominal_unit=V  v_nominal_value=1
      settings: SourceProductName=Simscape  SourceProductBaseCode=SS
  Redacted_2078 : PMIOPort  Side=Left
  Redacted_827 : PMIOPort  Port=2  Side=Left
  Redacted_65 : PMIOPort  Port=3  Side=Left
  Redacted_2555 : PMIOPort  Port=4  Side=Right
  Redacted_7416 : PMIOPort  Port=5  Side=Right
  connections:
  Redacted_827/RConn1 -- Redacted_7416/RConn1
  Redacted_2555/RConn1 -- Redacted_2078/RConn1
  Open Circuit/LConn1 -- Redacted_65/RConn1

== system Electrical_System_2018b_obfs/Redacted_1221/Redacted_7996/Redacted_7418/Redacted_4377/Redacted_6082/Redacted_2443/Redacted_6791 ==
  Redacted_497 : fl_lib/Electrical/Electrical Elements/Open Circuit  v_specify=off  v_priority=None  v=rijkoulpub V  v_nominal_specify=off  v_nominal_unit=V  v_nominal_value=whtojmaseb
      settings: SourceProductName=Simscape  SourceProductBaseCode=SS
  Redacted_2078 : PMIOPort  Side=Left
  Redacted_827 : PMIOPort  Port=2  Side=Left
  Redacted_65 : PMIOPort  Port=3  Side=Left
  Redacted_2555 : PMIOPort  Port=4  Side=Right
  Redacted_7416 : PMIOPort  Port=5  Side=Right
  connections:
  Redacted_7416/RConn1 -- Redacted_65/RConn1
  Redacted_2555/RConn1 -- Redacted_2078/RConn1
  Redacted_497/LConn1 -- Redacted_827/RConn1

== system Electrical_System_2018b_obfs/Redacted_1221/Redacted_7996/Redacted_7418/Redacted_4377/Redacted_6082/Redacted_248/Neutral_Negative ==
  Open Circuit : fl_lib/Electrical/Electrical Elements/Open Circuit  v_specify=off  v_priority=None  v=0 V  v_nominal_specify=off  v_nominal_unit=V  v_nominal_value=1
      settings: SourceProductName=Simscape  SourceProductBaseCode=SS
  Redacted_4518 : PMIOPort  Side=Left
  Redacted_7536 : PMIOPort  Port=2  Side=Left
  Redacted_9561 : PMIOPort  Port=3  Side=Left
  Redacted_1518 : PMIOPort  Port=4  Side=Right
  Redacted_7660 : PMIOPort  Port=5  Side=Right
  connections:
  Redacted_7536/RConn1 -- Redacted_1518/RConn1
  Open Circuit/LConn1 -- Redacted_4518/RConn1
  Redacted_7660/RConn1 -- Redacted_9561/RConn1

== system Electrical_System_2018b_obfs/Redacted_1221/Redacted_7996/Redacted_7418/Redacted_4377/Redacted_6082/Redacted_248/Positive_Neutral ==
  Open Circuit : fl_lib/Electrical/Electrical Elements/Open Circuit  v_specify=off  v_priority=None  v=0 V  v_nominal_specify=off  v_nominal_unit=V  v_nominal_value=1
      settings: SourceProductName=Simscape  SourceProductBaseCode=SS
  Redacted_4518 : PMIOPort  Side=Left
  Redacted_7536 : PMIOPort  Port=2  Side=Left
  Redacted_9561 : PMIOPort  Port=3  Side=Left
  Redacted_1518 : PMIOPort  Port=4  Side=Right
  Redacted_7660 : PMIOPort  Port=5  Side=Right
  connections:
  Redacted_7536/RConn1 -- Redacted_7660/RConn1
  Redacted_1518/RConn1 -- Redacted_4518/RConn1
  Open Circuit/LConn1 -- Redacted_9561/RConn1

== system Electrical_System_2018b_obfs/Redacted_1221/Redacted_7996/Redacted_7418/Redacted_4377/Redacted_6082/Redacted_248/Redacted_2281 ==
  Redacted_5475 : fl_lib/Electrical/Electrical Elements/Open Circuit  v_specify=off  v_priority=None  v=ayosrghose V  v_nominal_specify=off  v_nominal_unit=V  v_nominal_value=hotsbojhck
      settings: SourceProductName=Simscape  SourceProductBaseCode=SS
  Redacted_4518 : PMIOPort  Side=Left
  Redacted_7536 : PMIOPort  Port=2  Side=Left
  Redacted_9561 : PMIOPort  Port=3  Side=Left
  Redacted_1518 : PMIOPort  Port=4  Side=Right
  Redacted_7660 : PMIOPort  Port=5  Side=Right
  connections:
  Redacted_7660/RConn1 -- Redacted_9561/RConn1
  Redacted_1518/RConn1 -- Redacted_4518/RConn1
  Redacted_5475/LConn1 -- Redacted_7536/RConn1

== system Electrical_System_2018b_obfs/Redacted_1221/Redacted_7996/Redacted_7418/Redacted_4377/Redacted_6082/Redacted_2927/Neutral_Negative ==
  Open Circuit : fl_lib/Electrical/Electrical Elements/Open Circuit  v_specify=off  v_priority=None  v=0 V  v_nominal_specify=off  v_nominal_unit=V  v_nominal_value=1
      settings: SourceProductName=Simscape  SourceProductBaseCode=SS
  Redacted_7425 : PMIOPort  Side=Left
  Redacted_110 : PMIOPort  Port=2  Side=Left
  Redacted_9932 : PMIOPort  Port=3  Side=Left
  Redacted_5448 : PMIOPort  Port=4  Side=Right
  Redacted_18 : PMIOPort  Port=5  Side=Right
  connections:
  Redacted_18/RConn1 -- Redacted_9932/RConn1
  Open Circuit/LConn1 -- Redacted_7425/RConn1
  Redacted_110/RConn1 -- Redacted_5448/RConn1

== system Electrical_System_2018b_obfs/Redacted_1221/Redacted_7996/Redacted_7418/Redacted_4377/Redacted_6082/Redacted_2927/Positive_Neutral ==
  Open Circuit : fl_lib/Electrical/Electrical Elements/Open Circuit  v_specify=off  v_priority=None  v=0 V  v_nominal_specify=off  v_nominal_unit=V  v_nominal_value=1
      settings: SourceProductName=Simscape  SourceProductBaseCode=SS
  Redacted_7425 : PMIOPort  Side=Left
  Redacted_110 : PMIOPort  Port=2  Side=Left
  Redacted_9932 : PMIOPort  Port=3  Side=Left
  Redacted_5448 : PMIOPort  Port=4  Side=Right
  Redacted_18 : PMIOPort  Port=5  Side=Right
  connections:
  Open Circuit/LConn1 -- Redacted_9932/RConn1
  Redacted_5448/RConn1 -- Redacted_7425/RConn1
  Redacted_110/RConn1 -- Redacted_18/RConn1

== system Electrical_System_2018b_obfs/Redacted_1221/Redacted_7996/Redacted_7418/Redacted_4377/Redacted_6082/Redacted_2927/Redacted_9228 ==
  Redacted_5433 : fl_lib/Electrical/Electrical Elements/Open Circuit  v_specify=off  v_priority=None  v=mfngyahdfw V  v_nominal_specify=off  v_nominal_unit=V  v_nominal_value=hwwozmcwbx
      settings: SourceProductName=Simscape  SourceProductBaseCode=SS
  Redacted_7425 : PMIOPort  Side=Left
  Redacted_110 : PMIOPort  Port=2  Side=Left
  Redacted_9932 : PMIOPort  Port=3  Side=Left
  Redacted_5448 : PMIOPort  Port=4  Side=Right
  Redacted_18 : PMIOPort  Port=5  Side=Right
  connections:
  Redacted_5433/LConn1 -- Redacted_110/RConn1
  Redacted_5448/RConn1 -- Redacted_7425/RConn1
  Redacted_18/RConn1 -- Redacted_9932/RConn1

== system Electrical_System_2018b_obfs/Redacted_1221/Redacted_7996/Redacted_7418/Redacted_4377/Redacted_6082/Redacted_3086/Neutral_Negative ==
  Open Circuit : fl_lib/Electrical/Electrical Elements/Open Circuit  v_specify=off  v_priority=None  v=0 V  v_nominal_specify=off  v_nominal_unit=V  v_nominal_value=1
      settings: SourceProductName=Simscape  SourceProductBaseCode=SS
  Redacted_6054 : PMIOPort  Side=Left
  Redacted_5626 : PMIOPort  Port=2  Side=Left
  Redacted_6271 : PMIOPort  Port=3  Side=Left
  Redacted_2564 : PMIOPort  Port=4  Side=Right
  Redacted_7933 : PMIOPort  Port=5  Side=Right
  connections:
  Redacted_7933/RConn1 -- Redacted_6271/RConn1
  Open Circuit/LConn1 -- Redacted_6054/RConn1
  Redacted_5626/RConn1 -- Redacted_2564/RConn1

== system Electrical_System_2018b_obfs/Redacted_1221/Redacted_7996/Redacted_7418/Redacted_4377/Redacted_6082/Redacted_3086/Positive_Neutral ==
  Open Circuit : fl_lib/Electrical/Electrical Elements/Open Circuit  v_specify=off  v_priority=None  v=0 V  v_nominal_specify=off  v_nominal_unit=V  v_nominal_value=1
      settings: SourceProductName=Simscape  SourceProductBaseCode=SS
  Redacted_6054 : PMIOPort  Side=Left
  Redacted_5626 : PMIOPort  Port=2  Side=Left
  Redacted_6271 : PMIOPort  Port=3  Side=Left
  Redacted_2564 : PMIOPort  Port=4  Side=Right
  Redacted_7933 : PMIOPort  Port=5  Side=Right
  connections:
  Open Circuit/LConn1 -- Redacted_6271/RConn1
  Redacted_2564/RConn1 -- Redacted_6054/RConn1
  Redacted_5626/RConn1 -- Redacted_7933/RConn1
